simulink model "DVS2X_All_old"  (R2020b)
settings: Solver=VariableStepAuto  StartTime=0.0  StopTime=0.1  RelTol=1e-3
values from neighbouring files (symbols this model uses):
  k1 = 10^(gain/10)    (= 3.16227766017)    [LNA_tests.m]
  k3 = -4/3*(k1/vip3^2)    [LNA_tests.m]
  k5 = -(0.10875*k1+(3/4)*(vp1dB^2))*((8/5)*(1/vp1dB^4))    [LNA_tests.m]
  vip3 = sqrt(2*10^((IIP3-30)/10)*R)    [LNA_tests.m]
undefined symbols (not defined in the file or in its folder): dvbsapskmod
libraries: commutil2 x23, commdigbbndapm x20, dspsrcs4 x20, commfilt2 x20, commrflib2 x14, commchan3 x12, commsink2 x10, commrandsrc3 x10, commrfcorlib x7, commeq3 x5
(part 2 of 2)

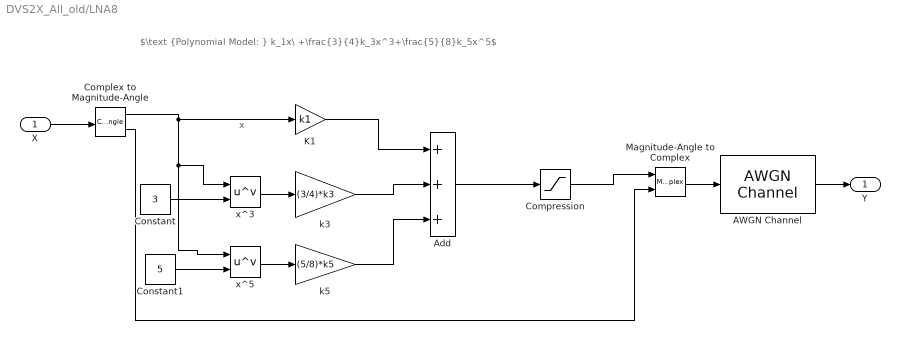
== system DVS2X_All_old/LNA8 ==
  note: x
  note: $\text {Polynomial Model: } k_1x\ +\frac{3}{4}k_3x^3+\frac{5}{8}k_5x^5$
  "X " : Inport
  AWGN Channel : commchan3/AWGN Channel  InputProcessing=Columns as channels (frame based)  seed=67  noiseMode="Signal to noise ratio  (Eb/No)"  EbNodB=23  EsNodB=10  SNRdB=10  bitsPerSym=4  Ps=1  Tsym=1e-6  variance=1
  Add : Sum  Inputs=+++
  Complex to Magnitude-Angle : ComplexToMagnitudeAngle
  "Compression " : Saturate  UpperLimit=2/3*vip3  LowerLimit=-1000
  Constant : Constant  Value=3
  Constant1 : Constant  Value=5
  K1 : Gain  Gain=k1
  Magnitude-Angle to Complex : MagnitudeAngleToComplex
  k3 : Gain  Gain=(3/4)*k3
  k5 : Gain  Gain=(5/8)*k5
  x^3 : Math  Operator=pow  SaturateOnIntegerOverflow=on
  x^5 : Math  Operator=pow  SaturateOnIntegerOverflow=on
  "Y " : Outport
  wires:
  Add/1 -> "Compression "/1
  Constant/1 -> x^3/2
  x^3/1 -> k3/1
  Constant1/1 -> x^5/2
  x^5/1 -> k5/1
  K1/1 -> Add/1
  k3/1 -> Add/2
  k5/1 -> Add/3
  "X "/1 -> Complex to Magnitude-Angle/1
  Complex to Magnitude-Angle/1 -> x^5/1, x^3/1, K1/1
  Complex to Magnitude-Angle/2 -> Magnitude-Angle to Complex/2
  "Compression "/1 -> Magnitude-Angle to Complex/1
  Magnitude-Angle to Complex/1 -> AWGN Channel/1
  AWGN Channel/1 -> "Y "/1
